simulink model "SixDOFSim"  (R2020b)
settings: Solver=VariableStepAuto  StartTime=0.0  StopTime=25  RelTol=1e-3
values from neighbouring files (symbols this model uses):
  A = q_d*S*CA    [nonlinear_6DOF.m]
  alpha_init = 0    [SixDOFModel.m]
  beta_init = 0    [SixDOFModel.m]
  eta_max = 10*pi/180    (= 0.174532925199)    [SixDOFModel.m]
  eta_min = - 25*pi/180    (= -0.436332312999)    [SixDOFModel.m]
  I_inv = inv(I)    [initializeParameters.m]
  K = place(A,B,ew_contr)    [SixDOFModel.m]
  m = 120000    [initializeParameters.m]
  Omega_init = [0;0;0]    [SixDOFModel.m]
  P_e_init = [100;0;-2000]    [SixDOFModel.m]
  Phi_init = [0;0;0]    [SixDOFModel.m]
  q = X(2)    [nonlinear_6DOF.m]
  r = X(5)    [nonlinear_6DOF.m]
  sigmaf_max = 10*pi/180    (= 0.174532925199)    [SixDOFModel.m]
  sigmaf_min = 0.5*pi/180    (= 0.00872664625997)    [SixDOFModel.m]
  U_test = [0.5;1;0;0]    [SixDOFModel.m]
  V_init = [20;0;0]    [SixDOFModel.m]
  vA_init = sqrt(V_init(1)^2+V_init(2)^2+V_init(3)^2)    [SixDOFModel.m]
  X_init = [alpha_init;Omega_init(2);vA_init;Phi_init(2);Omega_init(3);beta_init;Omega_init(1);Phi_init(1); P_e_init(1);P_e_init(2);P_e_init(3);Phi_init(3);V_init]    [SixDOFModel.m]
  xi_max = 25*pi/180    (= 0.436332312999)    [SixDOFModel.m]
  xi_min = - xi_max    (= -0.436332312999)    [SixDOFModel.m]
  zita_max = 30*pi/180    (= 0.523598775598)    [SixDOFModel.m]
  zita_min = - zita_max    (= -0.523598775598)    [SixDOFModel.m]
undefined symbols (not defined in the file or in its folder): B, Earth, F, Light, MIL, nonlinear_6DOF, WGS84
libraries: aerolibfltsims x5, aerolibtransform2 x4, aerolibwind2 x1, aerolibatmos2 x1
settings Model: Creator=teteu  LastModifiedBy=teteu
settings SolverCC: ZeroCrossAlgorithm=Adaptive
settings DebuggingCC: IgnoredZcDiagnostic=none

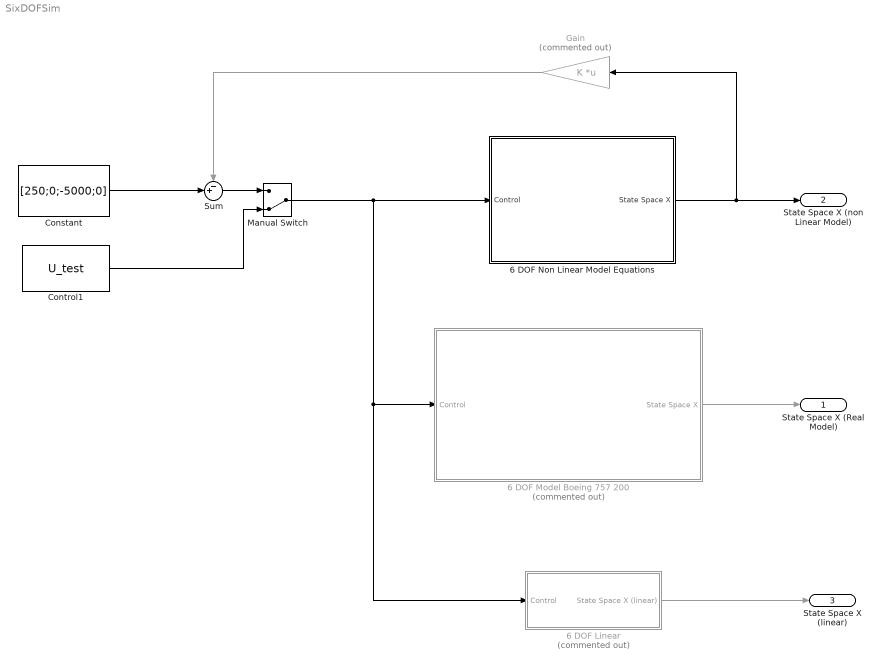
== system SixDOFSim ==
  6 DOF Linear : Subsystem  Commented=on
  6 DOF Model Boeing 757 200 : Subsystem  Commented=on
      mask Display: image('Eastern_Airlines_Boeing_757-225_N523EA_March_1990_DCW_4974892113-624x422.jpg'); % Use "Edit Image" on toolstrip to change.
  6 DOF Non Linear Model Equations : Subsystem
  Constant : Constant  Value=[250;0;-5000;0]
  Control1 : Constant  Value=U_test
  Gain : Gain  Commented=on  Gain=K  Multiplication=Matrix(K*u)
  Manual Switch : ManualSwitch  CurrentSetting=0
  Sum : Sum  Inputs=-+|
  State Space X (Real Model) : Outport
  State Space X (non Linear Model) : Outport  Port=2
  State Space X (linear) : Outport  Port=3
  wires:
  6 DOF Model Boeing 757 200/1(State Space X) -> State Space X (Real Model)/1
  6 DOF Non Linear Model Equations/1(State Space X) -> Gain/1, State Space X (non Linear Model)/1
  6 DOF Linear/1(State Space X (linear)) -> State Space X (linear)/1
  Gain/1 -> Sum/1
  Constant/1 -> Sum/2
  Sum/1 -> Manual Switch/1
  Control1/1 -> Manual Switch/2
  Manual Switch/1 -> 6 DOF Linear/1(Control), 6 DOF Model Boeing 757 200/1(Control), 6 DOF Non Linear Model Equations/1(Control)

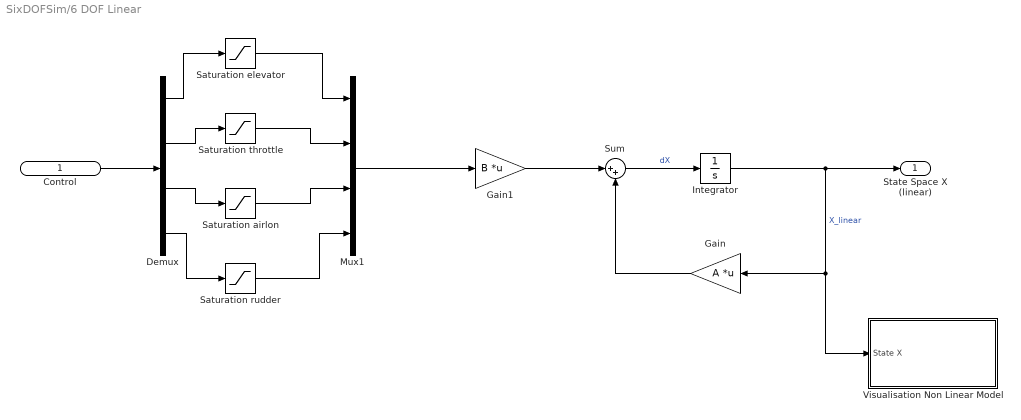
== system SixDOFSim/6 DOF Linear ==
  Control : Inport
  Demux : Demux
  Gain : Gain  Gain=A  Multiplication=Matrix(K*u)
  Gain1 : Gain  Gain=B  Multiplication=Matrix(K*u)
  Integrator : Integrator  InitialCondition=X_init
  Mux1 : Mux
  Saturation airlon : Saturate  UpperLimit=xi_max  LowerLimit=xi_min
  Saturation elevator : Saturate  UpperLimit=eta_max  LowerLimit=eta_min
  Saturation rudder : Saturate  UpperLimit=zita_max  LowerLimit=zita_min
  Saturation throttle : Saturate  UpperLimit=sigmaf_max  LowerLimit=sigmaf_min
  Sum : Sum  Inputs=|++
  Visualisation Non Linear Model : Subsystem
  State Space X (linear) : Outport
  wires:
  Gain1/1 -> Sum/1
  Integrator/1 -> State Space X (linear)/1, Visualisation Non Linear Model/1(State X), Gain/1  "X_linear"
  Mux1/1 -> Gain1/1
  Sum/1 -> Integrator/1  "dX"
  Gain/1 -> Sum/2
  Demux/2 -> Saturation throttle/1
  Demux/3 -> Saturation airlon/1
  Demux/1 -> Saturation elevator/1
  Control/1 -> Demux/1
  Saturation elevator/1 -> Mux1/1
  Saturation throttle/1 -> Mux1/2
  Saturation airlon/1 -> Mux1/3
  Saturation rudder/1 -> Mux1/4
  Demux/4 -> Saturation rudder/1

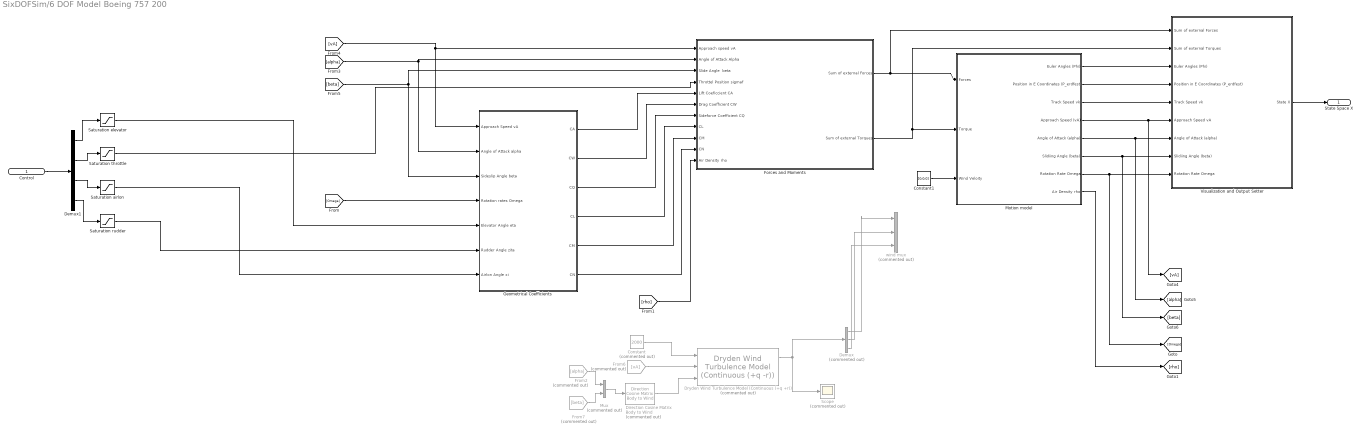
== system SixDOFSim/6 DOF Model Boeing 757 200 ==
  Control : Inport
  Constant : Constant  Commented=on  Value=2000
  Constant1 : Constant  Value=[0;0;0]
  Demux : Demux  Commented=on  Outputs=3
  Demux1 : Demux
  Direction Cosine Matrix Body to Wind : aerolibtransform2/Direction Cosine Matrix Body to Wind  Commented=on
      settings: SourceProductBaseCode=AE
  Dryden Wind Turbulence Model (Continuous (+q +r)) : aerolibwind2/Dryden Wind Turbulence Model  (Continuous (+q -r))  Commented=on  units=Metric (MKS)  spec=MIL-F-8785C  model=Continuous Dryden (+q +r)  W20=15  Wdeg=0  TurbProb=10^-2 - Light  L_high=533.4  Wingspan=10  ts=0.1  Seed=[23341 23342 23343 23344]  T_on=on
  Forces and Moments : Subsystem
  From2 : From  Commented=on  GotoTag=alpha
  From6 : From  Commented=on  GotoTag=vA
  From7 : From  Commented=on  GotoTag=beta
  Geometrical Coefficients : Subsystem
  "Motion model " : Subsystem
  Mux : Mux  Commented=on  Inputs=2
  Saturation airlon : Saturate  UpperLimit=xi_max  LowerLimit=xi_min
  Saturation elevator : Saturate  UpperLimit=eta_max  LowerLimit=eta_min
  Saturation rudder : Saturate  UpperLimit=zita_max  LowerLimit=zita_min
  Saturation throttle : Saturate  UpperLimit=sigmaf_max  LowerLimit=sigmaf_min
  Scope : Scope  Commented=on
  Visualization and Output Setter : Subsystem
  wind mux : Mux  Commented=on  Inputs=3
  State Space X : Outport
  wires:
  "Motion model "/7(Rotation Rate Omega) -> [Omega], Visualization and Output Setter/9(Rotation Rate Omega)
  "Motion model "/3(Track Speed vk) -> Visualization and Output Setter/5(Track Speed vk)
  Dryden Wind Turbulence Model (Continuous (+q +r))/1 -> Scope/1, Demux/1
  Visualization and Output Setter/1(State X) -> State Space X/1
  "Motion model "/6(Slidiing Angle (beta)) -> [beta], Visualization and Output Setter/8(Slidiing Angle (beta))
  Forces and Moments/2(Sum of external Torques) -> "Motion model "/2(Torque), Visualization and Output Setter/2(Sum of external Torques)
  [alpha] -> Geometrical Coefficients/2(Angle of Attack alpha), Forces and Moments/2(Angle of Attack Alpha)
  "Motion model "/4(Approach Speed (vA)) -> [vA], Visualization and Output Setter/6(Approach Speed vA)
  Geometrical Coefficients/4(CL) -> Forces and Moments/8(CL)
  Geometrical Coefficients/1(CA) -> Forces and Moments/5(Lift Coeficcient CA)
  Forces and Moments/1(Sum of external Forces) -> Visualization and Output Setter/1(Sum of external Forces), "Motion model "/1(Forces)
  "Motion model "/5(Angle of Attack (alpha)) -> [alpha], Visualization and Output Setter/7(Angle of Attack (alpha))
  "Motion model "/2(Position in E Coordinates (P_erdfest)) -> Visualization and Output Setter/4(Position in E Coordinates (P_erdfest))
  "Motion model "/1(Euler Angles (Phi)) -> Visualization and Output Setter/3(Euler Angles (Phi))
  [vA] -> Geometrical Coefficients/1(Approach Speed vA), Forces and Moments/1(Approach speed vA)
  Geometrical Coefficients/5(CM) -> Forces and Moments/9(CM)
  Saturation airlon/1 -> Geometrical Coefficients/7(Airlon Angle xi)
  [Omega] -> Geometrical Coefficients/4(Rotation rates Omega)
  Saturation throttle/1 -> Forces and Moments/4(Throttel Position sigmaf)
  [beta] -> Geometrical Coefficients/3(Sideslip Angle beta), Forces and Moments/3(Slide Angle  beta)
  Geometrical Coefficients/6(CN) -> Forces and Moments/10(CN)
  "Motion model "/8(Air Density rho) -> [rho]
  [rho] -> Forces and Moments/11(Air Density rho)
  Saturation elevator/1 -> Geometrical Coefficients/5(Elevator Angle eta)
  Saturation rudder/1 -> Geometrical Coefficients/6(Rudder Angle zita)
  Geometrical Coefficients/3(CQ) -> Forces and Moments/7(Sideforce Coefficient CQ)
  Constant/1 -> Dryden Wind Turbulence Model (Continuous (+q +r))/1
  Geometrical Coefficients/2(CW) -> Forces and Moments/6(Drag Coefficient CW)
  From6/1 -> Dryden Wind Turbulence Model (Continuous (+q +r))/2
  Demux/1 -> wind mux/1
  Demux/2 -> wind mux/2
  Demux/3 -> wind mux/3
  Direction Cosine Matrix Body to Wind/1 -> Dryden Wind Turbulence Model (Continuous (+q +r))/3
  From2/1 -> Mux/1
  From7/1 -> Mux/2
  Mux/1 -> Direction Cosine Matrix Body to Wind/1
  Constant1/1 -> "Motion model "/3(Wind Veloity)
  Demux1/2 -> Saturation throttle/1
  Demux1/3 -> Saturation airlon/1
  Demux1/1 -> Saturation elevator/1
  Control/1 -> Demux1/1
  Demux1/4 -> Saturation rudder/1

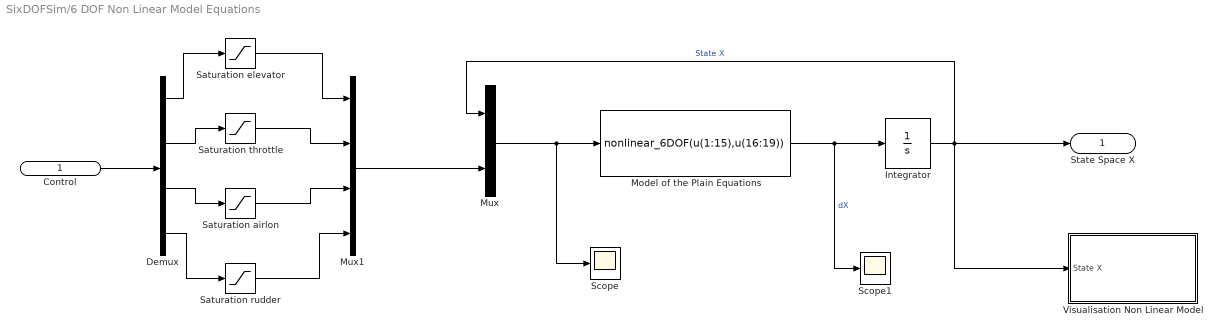
== system SixDOFSim/6 DOF Non Linear Model Equations ==
  Control : Inport
  Demux : Demux
  Integrator : Integrator  InitialCondition=X_init
  Model of the Plain Equations : MATLABFcn  MATLABFcn=nonlinear_6DOF(u(1:15),u(16:19))
  Mux : Mux  Inputs=2
  Mux1 : Mux
  Saturation airlon : Saturate  UpperLimit=xi_max  LowerLimit=xi_min
  Saturation elevator : Saturate  UpperLimit=eta_max  LowerLimit=eta_min
  Saturation rudder : Saturate  UpperLimit=zita_max  LowerLimit=zita_min
  Saturation throttle : Saturate  UpperLimit=sigmaf_max  LowerLimit=sigmaf_min
  Scope : Scope
  Scope1 : Scope
  Visualisation Non Linear Model : Subsystem
  State Space X : Outport
  wires:
  Model of the Plain Equations/1 -> Scope1/1, Integrator/1  "dX"
  Integrator/1 -> State Space X/1, Visualisation Non Linear Model/1(State X), Mux/1  "State X"
  Mux/1 -> Scope/1, Model of the Plain Equations/1
  Demux/1 -> Saturation elevator/1
  Demux/2 -> Saturation throttle/1
  Demux/3 -> Saturation airlon/1
  Demux/4 -> Saturation rudder/1
  Saturation elevator/1 -> Mux1/1
  Saturation throttle/1 -> Mux1/2
  Saturation airlon/1 -> Mux1/3
  Saturation rudder/1 -> Mux1/4
  Mux1/1 -> Mux/2
  Control/1 -> Demux/1

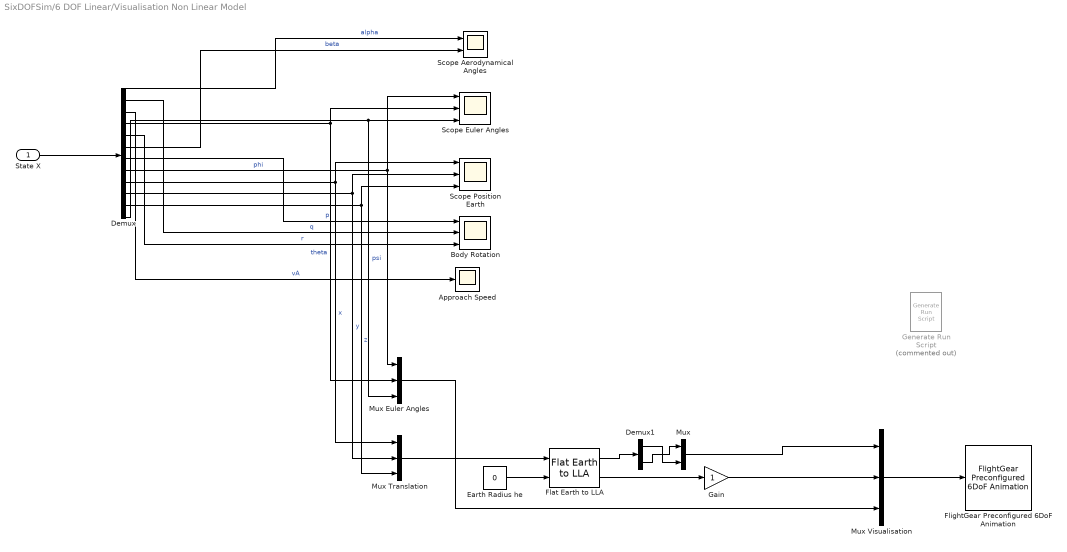
== system SixDOFSim/6 DOF Linear/Visualisation Non Linear Model ==
  State X : Inport
  Approach Speed : Scope
  Body Rotation : Scope  NumInputPorts=3
  Demux : Demux  Outputs=12
  Demux1 : Demux  Outputs=2
  Earth Radius he : Constant  Value=0
  Flat Earth to LLA : aerolibtransform2/Flat Earth to LLA  units=Metric (MKS)  ptype=Earth (WGS84)  F=1/298.257223563  R=6378137  refPosPort=off  LL0=[0 10]  psi=0
  FlightGear Preconfigured 6DoF Animation : aerolibfltsims/FlightGear Preconfigured 6DoF Animation  xFlightGearVersion=v2019.1  DestinationIpAddress=127.0.0.1  DestinationPort=5502  SampleTime=1/30  packetVersion=24
  Gain : Gain
  Generate Run Script : aerolibfltsims/Generate Run Script  Commented=on  Architecture=Win64  dataFlow=Send  GeometryModelName=c172p  AirportId=KSFO  RunwayId=10L  InitialAltitude=7224  InitialHeading=113  OffsetDistance=4.72  OffsetAzimuth=0  InstallScenery=off  DisableShaders=on  OriginAddress=127.0.0.1  DestinationPort=5502  OriginPort=5505  LocalAddress=127.0.0.1  OutputFileName=runfg.bat  FlightGearBaseDirectory=D:\Flight Gear\FlightGear 2018.1.1
  Mux : Mux  Inputs=2
  Mux Euler Angles : Mux  Inputs=3
  "Mux Translation " : Mux  Inputs=3
  Mux Visualisation : Mux  Inputs=3
  Scope Aerodynamical Angles : Scope  NumInputPorts=2
  Scope Euler Angles : Scope  NumInputPorts=3
  Scope Position Earth : Scope  NumInputPorts=3
  wires:
  Demux/4 -> Mux Euler Angles/2, Scope Euler Angles/2  "theta"
  Demux/10 -> Scope Position Earth/2, "Mux Translation "/2  "y"
  Demux/7 -> Body Rotation/1  "p"
  Demux/12 -> Scope Euler Angles/3, Mux Euler Angles/3  "psi"
  Demux/9 -> "Mux Translation "/1, Scope Position Earth/1  "x"
  Demux/8 -> Mux Euler Angles/1, Scope Euler Angles/1  "phi"
  Demux/6 -> Scope Aerodynamical Angles/2  "beta"
  Demux/3 -> Approach Speed/1  "vA"
  Demux/11 -> Scope Position Earth/3, "Mux Translation "/3  "z"
  Demux/1 -> Scope Aerodynamical Angles/1  "alpha"
  Demux/2 -> Body Rotation/2  "q"
  Demux/5 -> Body Rotation/3  "r"
  State X/1 -> Demux/1
  Earth Radius he/1 -> Flat Earth to LLA/2
  "Mux Translation "/1 -> Flat Earth to LLA/1
  Mux Visualisation/1 -> FlightGear Preconfigured 6DoF Animation/1
  Flat Earth to LLA/1 -> Demux1/1
  Demux1/1 -> Mux/2
  Demux1/2 -> Mux/1
  Mux/1 -> Mux Visualisation/1
  Mux Euler Angles/1 -> Mux Visualisation/3
  Gain/1 -> Mux Visualisation/2
  Flat Earth to LLA/2 -> Gain/1

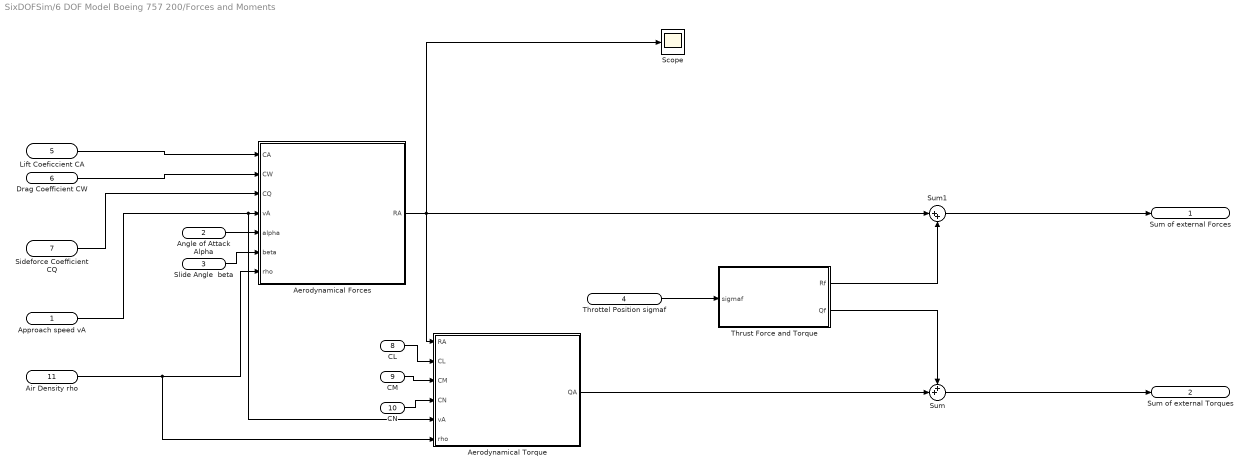
== system SixDOFSim/6 DOF Model Boeing 757 200/Forces and Moments ==
  Approach speed vA : Inport
  Angle of Attack Alpha : Inport  Port=2
  Slide Angle  beta : Inport  Port=3
  Throttel Position sigmaf : Inport  Port=4
  Lift Coeficcient CA : Inport  Port=5
  Drag Coefficient CW : Inport  Port=6
  Sideforce Coefficient CQ : Inport  Port=7
  CL : Inport  Port=8
  CM : Inport  Port=9
  CN : Inport  Port=10
  Air Density rho : Inport  Port=11
  Aerodynamical Forces : MATLAB Function  TreatAsAtomicUnit=on
  Aerodynamical Torque : MATLAB Function  TreatAsAtomicUnit=on
  Scope : Scope
  Sum : Sum  Inputs=++|
  Sum1 : Sum  Inputs=|++
  Thrust Force and Torque : MATLAB Function  TreatAsAtomicUnit=on
  Sum of external Forces : Outport
  Sum of external Torques : Outport  Port=2
  wires:
  Aerodynamical Forces/1(RA) -> Scope/1, Sum1/1, Aerodynamical Torque/1(RA)
  Aerodynamical Torque/1(QA) -> Sum/2
  Sum1/1 -> Sum of external Forces/1
  Sum/1 -> Sum of external Torques/1
  Throttel Position sigmaf/1 -> Thrust Force and Torque/1(sigmaf)
  Thrust Force and Torque/1(Rf) -> Sum1/2
  Thrust Force and Torque/2(Qf) -> Sum/1
  Angle of Attack Alpha/1 -> Aerodynamical Forces/5(alpha)
  Slide Angle  beta/1 -> Aerodynamical Forces/6(beta)
  Approach speed vA/1 -> Aerodynamical Torque/5(vA), Aerodynamical Forces/4(vA)
  Lift Coeficcient CA/1 -> Aerodynamical Forces/1(CA)
  Drag Coefficient CW/1 -> Aerodynamical Forces/2(CW)
  Sideforce Coefficient CQ/1 -> Aerodynamical Forces/3(CQ)
  CL/1 -> Aerodynamical Torque/2(CL)
  CM/1 -> Aerodynamical Torque/3(CM)
  CN/1 -> Aerodynamical Torque/4(CN)
  Air Density rho/1 -> Aerodynamical Torque/6(rho), Aerodynamical Forces/7(rho)

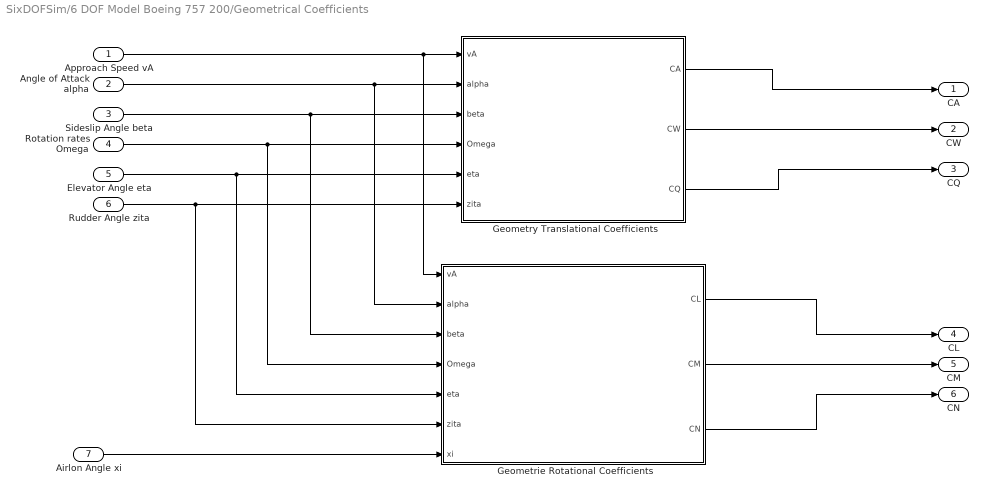
== system SixDOFSim/6 DOF Model Boeing 757 200/Geometrical Coefficients ==
  Approach Speed vA : Inport
  Angle of Attack alpha : Inport  Port=2
  Sideslip Angle beta : Inport  Port=3
  Rotation rates Omega : Inport  Port=4
  Elevator Angle eta : Inport  Port=5
  Rudder Angle zita : Inport  Port=6
  Airlon Angle xi : Inport  Port=7
  Geometrie Rotational Coefficients : MATLAB Function  TreatAsAtomicUnit=on
  Geometry Translational Coefficients : MATLAB Function  TreatAsAtomicUnit=on
  CA : Outport
  CW : Outport  Port=2
  CQ : Outport  Port=3
  CL : Outport  Port=4
  CM : Outport  Port=5
  CN : Outport  Port=6
  wires:
  Elevator Angle eta/1 -> Geometrie Rotational Coefficients/5(eta), Geometry Translational Coefficients/5(eta)
  Angle of Attack alpha/1 -> Geometrie Rotational Coefficients/2(alpha), Geometry Translational Coefficients/2(alpha)
  Geometrie Rotational Coefficients/1(CL) -> CL/1
  Geometry Translational Coefficients/3(CQ) -> CQ/1
  Geometrie Rotational Coefficients/3(CN) -> CN/1
  Approach Speed vA/1 -> Geometrie Rotational Coefficients/1(vA), Geometry Translational Coefficients/1(vA)
  Geometry Translational Coefficients/1(CA) -> CA/1
  Sideslip Angle beta/1 -> Geometrie Rotational Coefficients/3(beta), Geometry Translational Coefficients/3(beta)
  Rudder Angle zita/1 -> Geometrie Rotational Coefficients/6(zita), Geometry Translational Coefficients/6(zita)
  Geometry Translational Coefficients/2(CW) -> CW/1
  Rotation rates Omega/1 -> Geometrie Rotational Coefficients/4(Omega), Geometry Translational Coefficients/4(Omega)
  Geometrie Rotational Coefficients/2(CM) -> CM/1
  Airlon Angle xi/1 -> Geometrie Rotational Coefficients/7(xi)

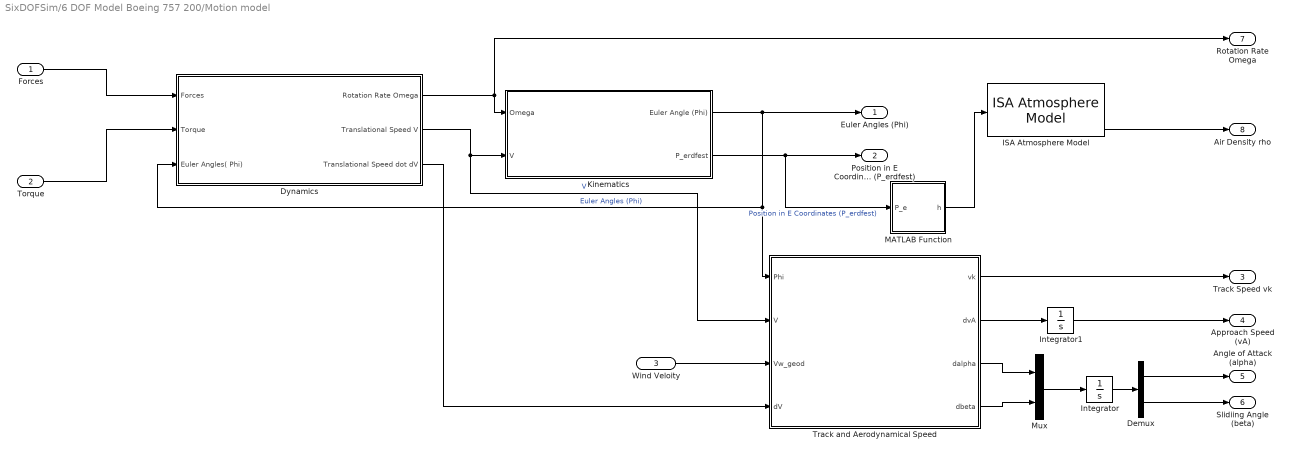
== system SixDOFSim/6 DOF Model Boeing 757 200/Motion model  ==
  Forces : Inport
  Torque : Inport  Port=2
  Wind Veloity : Inport  Port=3
  Demux : Demux  Outputs=2
  Dynamics : Subsystem
  ISA Atmosphere Model : aerolibatmos2/ISA Atmosphere Model  custom=off  g=9.80665  gamma=1.4  R=287.0531  L=0.0065  h_trop=11000  h_strat=20000  rho0=1.225  P0=101325  T0=288.15  h0=0
  Integrator : Integrator  InitialCondition=[alpha_init;beta_init]
  Integrator1 : Integrator  InitialCondition=vA_init
  Kinematics : Subsystem
  MATLAB Function : MATLAB Function  TreatAsAtomicUnit=on
  Mux : Mux  Inputs=2
  Track and Aerodynamical Speed : MATLAB Function  TreatAsAtomicUnit=on
  Euler Angles (Phi) : Outport
  Position in E Coordinates (P_erdfest) : Outport  Port=2
  Track Speed vk : Outport  Port=3
  Approach Speed (vA) : Outport  Port=4
  Angle of Attack (alpha) : Outport  Port=5
  Slidiing Angle (beta) : Outport  Port=6
  Rotation Rate Omega : Outport  Port=7
  Air Density rho : Outport  Port=8
  wires:
  Torque/1 -> Dynamics/2(Torque)
  Kinematics/1(Euler Angle (Phi)) -> Track and Aerodynamical Speed/1(Phi), Dynamics/3(Euler Angles( Phi)), Euler Angles (Phi)/1  "Euler Angles (Phi)"
  Kinematics/2(P_erdfest) -> Position in E Coordinates (P_erdfest)/1, MATLAB Function/1(P_e)  "Position in E Coordinates (P_erdfest)"
  Dynamics/2(Translational Speed V) -> Track and Aerodynamical Speed/2(V), Kinematics/2(V)  "V"
  Forces/1 -> Dynamics/1(Forces)
  Dynamics/1(Rotation Rate Omega) -> Kinematics/1(Omega), Rotation Rate Omega/1
  Wind Veloity/1 -> Track and Aerodynamical Speed/3(Vw_geod)
  MATLAB Function/1(h) -> ISA Atmosphere Model/1
  ISA Atmosphere Model/4 -> Air Density rho/1
  Track and Aerodynamical Speed/1(vk) -> Track Speed vk/1
  Dynamics/3(Translational Speed dot dV) -> Track and Aerodynamical Speed/4(dV)
  Mux/1 -> Integrator/1
  Integrator/1 -> Demux/1
  Demux/1 -> Angle of Attack (alpha)/1
  Demux/2 -> Slidiing Angle (beta)/1
  Track and Aerodynamical Speed/3(dalpha) -> Mux/1
  Track and Aerodynamical Speed/4(dbeta) -> Mux/2
  Track and Aerodynamical Speed/2(dvA) -> Integrator1/1
  Integrator1/1 -> Approach Speed (vA)/1

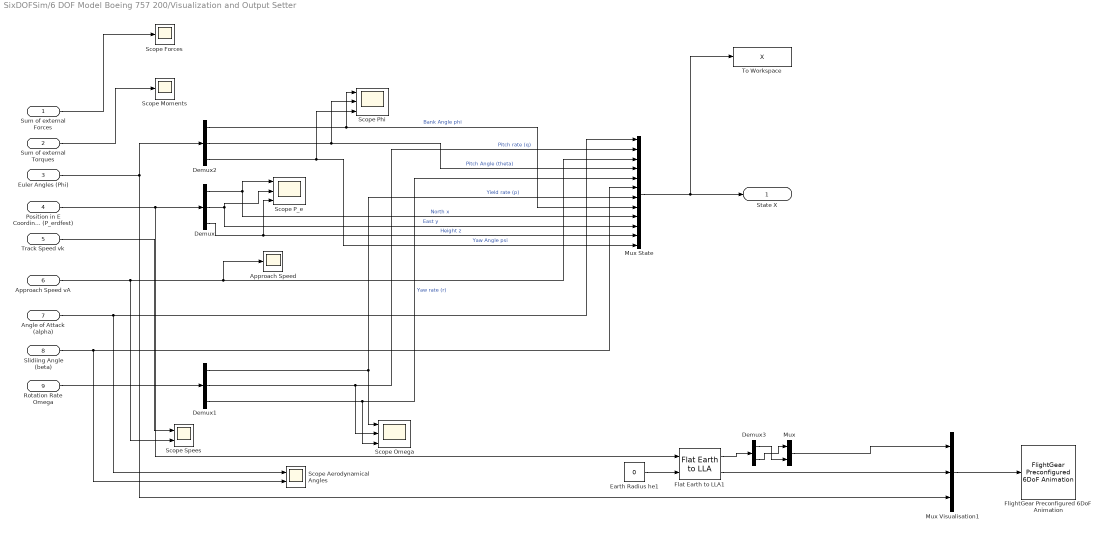
== system SixDOFSim/6 DOF Model Boeing 757 200/Visualization and Output Setter ==
  Sum of external Forces : Inport
  Sum of external Torques : Inport  Port=2
  Euler Angles (Phi) : Inport  Port=3
  Position in E Coordinates (P_erdfest) : Inport  Port=4
  Track Speed vk : Inport  Port=5
  Approach Speed vA : Inport  Port=6
  Angle of Attack (alpha) : Inport  Port=7
  Slidiing Angle (beta) : Inport  Port=8
  Rotation Rate Omega : Inport  Port=9
  Approach Speed : Scope
  Demux : Demux  Outputs=3
  Demux1 : Demux  Outputs=3
  Demux2 : Demux  Outputs=3
  Demux3 : Demux  Outputs=2
  Earth Radius he1 : Constant  Value=0
  Flat Earth to LLA1 : aerolibtransform2/Flat Earth to LLA  units=Metric (MKS)  ptype=Earth (WGS84)  F=1/298.257223563  R=6378137  refPosPort=off  LL0=[0 10]  psi=0
  FlightGear Preconfigured 6DoF Animation : aerolibfltsims/FlightGear Preconfigured 6DoF Animation  xFlightGearVersion=v2019.1  DestinationIpAddress=127.0.0.1  DestinationPort=5502  SampleTime=1/30  packetVersion=24
  Mux : Mux  Inputs=2
  Mux State : Mux  Inputs=12
  Mux Visualisation1 : Mux  Inputs=3
  Scope Aerodynamical Angles : Scope  NumInputPorts=2
  Scope Forces : Scope
  Scope Moments : Scope
  Scope Omega : Scope  NumInputPorts=3
  Scope P_e : Scope  NumInputPorts=3
  Scope Phi : Scope  NumInputPorts=3
  Scope Spees : Scope  NumInputPorts=2
  To Workspace : ToWorkspace  VariableName=X  SaveFormat=Timeseries  SampleTime=-1
  State X : Outport
  wires:
  Rotation Rate Omega/1 -> Demux1/1
  Position in E Coordinates (P_erdfest)/1 -> Demux/1, Flat Earth to LLA1/1
  Mux State/1 -> To Workspace/1, State X/1
  Angle of Attack (alpha)/1 -> Mux State/1, Scope Aerodynamical Angles/1
  Demux1/2 -> Mux State/2, Scope Omega/2  "Pitch rate (q)"
  Approach Speed vA/1 -> Scope Spees/2, Approach Speed/1, Mux State/3
  Euler Angles (Phi)/1 -> Demux2/1, Mux Visualisation1/3
  Demux2/2 -> Mux State/4, Scope Phi/2  "Pitch Angle (theta)"
  Demux1/3 -> Mux State/5, Scope Omega/3  "Yaw rate (r)"
  Slidiing Angle (beta)/1 -> Mux State/6, Scope Aerodynamical Angles/2
  Demux1/1 -> Scope Omega/1, Mux State/7  "Yield rate (p)"
  Demux2/1 -> Scope Phi/1, Mux State/8  "Bank Angle phi"
  Demux/1 -> Scope P_e/1, Mux State/9  "North x"
  Demux/2 -> Scope P_e/2, Mux State/10  "East y"
  Demux/3 -> Scope P_e/3, Mux State/11  "Height z"
  Demux2/3 -> Mux State/12, Scope Phi/3  "Yaw Angle psi"
  Sum of external Forces/1 -> Scope Forces/1
  Sum of external Torques/1 -> Scope Moments/1
  Track Speed vk/1 -> Scope Spees/1
  Demux3/1 -> Mux/2
  Flat Earth to LLA1/2 -> Mux Visualisation1/2
  Demux3/2 -> Mux/1
  Mux Visualisation1/1 -> FlightGear Preconfigured 6DoF Animation/1
  Flat Earth to LLA1/1 -> Demux3/1
  Earth Radius he1/1 -> Flat Earth to LLA1/2
  Mux/1 -> Mux Visualisation1/1

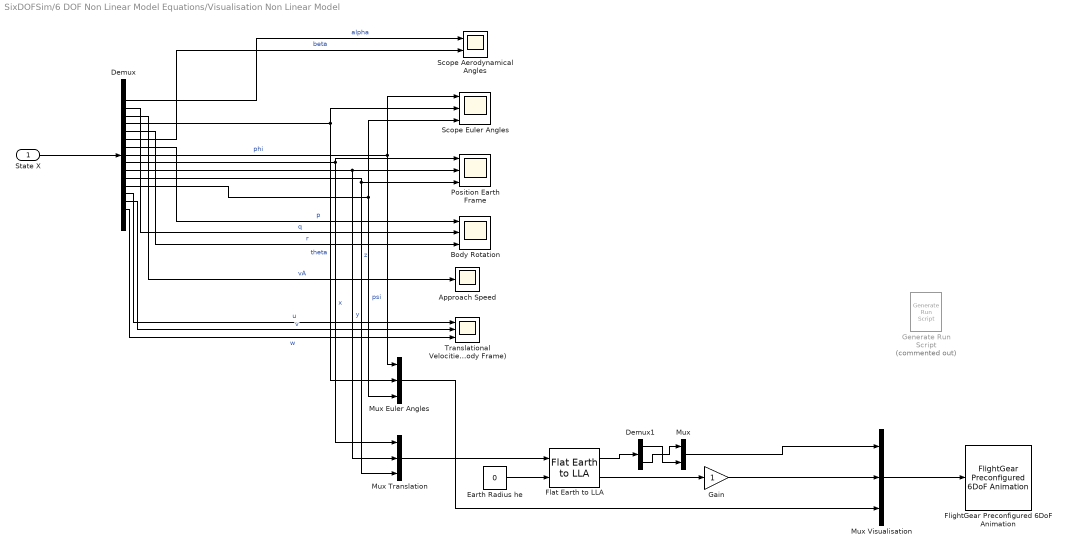
== system SixDOFSim/6 DOF Non Linear Model Equations/Visualisation Non Linear Model ==
  State X : Inport
  Approach Speed : Scope
  Body Rotation : Scope  NumInputPorts=3
  Demux : Demux  Outputs=15
  Demux1 : Demux  Outputs=2
  Earth Radius he : Constant  Value=0
  Flat Earth to LLA : aerolibtransform2/Flat Earth to LLA  units=Metric (MKS)  ptype=Earth (WGS84)  F=1/298.257223563  R=6378137  refPosPort=off  LL0=[0 10]  psi=0
  FlightGear Preconfigured 6DoF Animation : aerolibfltsims/FlightGear Preconfigured 6DoF Animation  xFlightGearVersion=v2019.1  DestinationIpAddress=127.0.0.1  DestinationPort=5502  SampleTime=1/30  packetVersion=24
  Gain : Gain
  Generate Run Script : aerolibfltsims/Generate Run Script  Commented=on  Architecture=Win64  dataFlow=Send  GeometryModelName=c172p  AirportId=KSFO  RunwayId=10L  InitialAltitude=7224  InitialHeading=113  OffsetDistance=4.72  OffsetAzimuth=0  InstallScenery=off  DisableShaders=on  OriginAddress=127.0.0.1  DestinationPort=5502  OriginPort=5505  LocalAddress=127.0.0.1  OutputFileName=runfg.bat  FlightGearBaseDirectory=D:\Flight Gear\FlightGear 2018.1.1
  Mux : Mux  Inputs=2
  Mux Euler Angles : Mux  Inputs=3
  "Mux Translation " : Mux  Inputs=3
  Mux Visualisation : Mux  Inputs=3
  Position Earth Frame : Scope  NumInputPorts=3
  Scope Aerodynamical Angles : Scope  NumInputPorts=2
  Scope Euler Angles : Scope  NumInputPorts=3
  Translational Velocities (Body Frame) : Scope  NumInputPorts=3
  wires:
  Demux/4 -> Mux Euler Angles/2, Scope Euler Angles/2  "theta"
  Demux/10 -> "Mux Translation "/2, Position Earth Frame/2  "y"
  Demux/7 -> Body Rotation/1  "p"
  Demux/12 -> Scope Euler Angles/3, Mux Euler Angles/3  "psi"
  Demux/9 -> "Mux Translation "/1, Position Earth Frame/1  "x"
  Demux/8 -> Mux Euler Angles/1, Scope Euler Angles/1  "phi"
  Demux/6 -> Scope Aerodynamical Angles/2  "beta"
  Demux/3 -> Approach Speed/1  "vA"
  Demux/11 -> "Mux Translation "/3, Position Earth Frame/3  "z"
  Demux/1 -> Scope Aerodynamical Angles/1  "alpha"
  Demux/2 -> Body Rotation/2  "q"
  Demux/5 -> Body Rotation/3  "r"
  State X/1 -> Demux/1
  Earth Radius he/1 -> Flat Earth to LLA/2
  "Mux Translation "/1 -> Flat Earth to LLA/1
  Mux Visualisation/1 -> FlightGear Preconfigured 6DoF Animation/1
  Flat Earth to LLA/1 -> Demux1/1
  Demux1/1 -> Mux/2
  Demux1/2 -> Mux/1
  Mux/1 -> Mux Visualisation/1
  Mux Euler Angles/1 -> Mux Visualisation/3
  Gain/1 -> Mux Visualisation/2
  Flat Earth to LLA/2 -> Gain/1
  Demux/13 -> Translational Velocities (Body Frame)/1  "u"
  Demux/14 -> Translational Velocities (Body Frame)/2  "v"
  Demux/15 -> Translational Velocities (Body Frame)/3  "w"

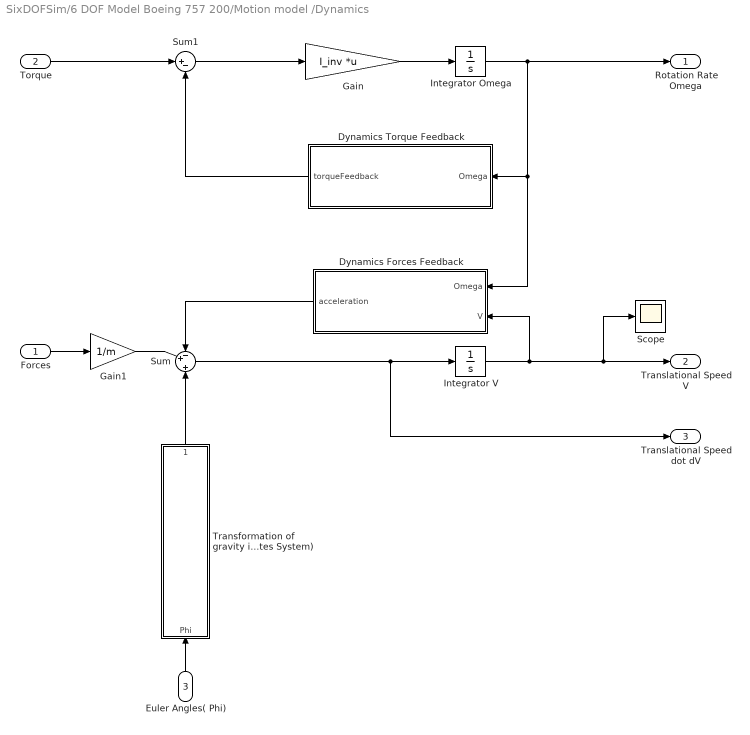
== system SixDOFSim/6 DOF Model Boeing 757 200/Motion model /Dynamics ==
  Forces : Inport
  Torque : Inport  Port=2
  Euler Angles( Phi) : Inport  Port=3
  Dynamics Forces Feedback : MATLAB Function  TreatAsAtomicUnit=on
  Dynamics Torque Feedback : MATLAB Function  TreatAsAtomicUnit=on
  Gain : Gain  Gain=I_inv  Multiplication=Matrix(K*u) (u vector)
  Gain1 : Gain  Gain=1/m
  Integrator Omega : Integrator  InitialCondition=Omega_init
  Integrator V : Integrator  InitialCondition=V_init
  Scope : Scope
  Sum : Sum  Inputs=-+|+
  Sum1 : Sum  Inputs=|+-
  Transformation of gravity in (Körperfestes System) : MATLAB Function  TreatAsAtomicUnit=on
  Rotation Rate Omega : Outport
  Translational Speed V : Outport  Port=2
  Translational Speed dot dV : Outport  Port=3
  wires:
  Euler Angles( Phi)/1 -> Transformation of gravity in (Körperfestes System)/1(Phi)
  Transformation of gravity in (Körperfestes System)/1(gravityAcceleration) -> Sum/3
  Forces/1 -> Gain1/1
  Sum/1 -> Translational Speed dot dV/1, Integrator V/1
  Integrator V/1 -> Scope/1, Translational Speed V/1, Dynamics Forces Feedback/2(V)
  Gain1/1 -> Sum/2
  Dynamics Forces Feedback/1(acceleration) -> Sum/1
  Torque/1 -> Sum1/1
  Sum1/1 -> Gain/1
  Gain/1 -> Integrator Omega/1
  Integrator Omega/1 -> Dynamics Forces Feedback/1(Omega), Dynamics Torque Feedback/1(Omega), Rotation Rate Omega/1
  Dynamics Torque Feedback/1(torqueFeedback) -> Sum1/2

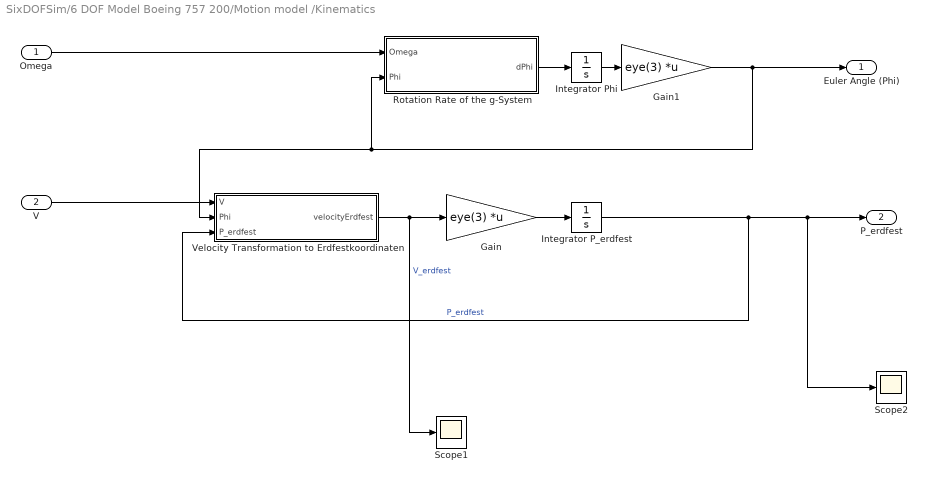
== system SixDOFSim/6 DOF Model Boeing 757 200/Motion model /Kinematics ==
  Omega : Inport
  V : Inport  Port=2
  Gain : Gain  Gain=eye(3)  Multiplication=Matrix(K*u) (u vector)
  Gain1 : Gain  Gain=eye(3)  Multiplication=Matrix(K*u) (u vector)
  Integrator P_erdfest : Integrator  InitialCondition=P_e_init
  Integrator Phi : Integrator  InitialCondition=Phi_init
  Rotation Rate of the g-System : MATLAB Function  TreatAsAtomicUnit=on
  Scope1 : Scope
  Scope2 : Scope
  Velocity Transformation to Erdfestkoordinaten : MATLAB Function  TreatAsAtomicUnit=on
  Euler Angle (Phi) : Outport
  P_erdfest : Outport  Port=2
  wires:
  Integrator P_erdfest/1 -> Scope2/1, P_erdfest/1, Velocity Transformation to Erdfestkoordinaten/3(P_erdfest)  "P_erdfest"
  Velocity Transformation to Erdfestkoordinaten/1(velocityErdfest) -> Scope1/1, Gain/1  "V_erdfest"
  V/1 -> Velocity Transformation to Erdfestkoordinaten/1(V)
  Rotation Rate of the g-System/1(dPhi) -> Integrator Phi/1
  Gain/1 -> Integrator P_erdfest/1
  Omega/1 -> Rotation Rate of the g-System/1(Omega)
  Integrator Phi/1 -> Gain1/1
  Gain1/1 -> Rotation Rate of the g-System/2(Phi), Velocity Transformation to Erdfestkoordinaten/2(Phi), Euler Angle (Phi)/1

== matlab function SixDOFSim/6 DOF Model Boeing 757 200/Motion model /Dynamics/Transformation of gravity in (Körperfestes System) ==
  data: Phi input; gravityAcceleration output; g parameter
function gravityAcceleration = Tfg(Phi,g)
G_geod = [0;0;g]; %Graviation vector in geodetic ref. Frame
Tfg = coordTransfMatrix(Phi(1),1)*coordTransfMatrix(Phi(2),2)*coordTransfMatrix(Phi(3),3); % Transformation Matrix goedetic --> body reference Frame
gravityAcceleration = Tfg*G_geod;

== matlab function SixDOFSim/6 DOF Model Boeing 757 200/Motion model /Kinematics/Rotation Rate of the g-System ==
  data: Omega input; dPhi output; Phi input
function dPhi = J(Omega,Phi)
%Rotation rate of the g-system depending on the euler angles
%Phi: euler Angles
%Omega_ diff = Omega-Omega_g
%dPhi: Rotaion Speed considering the rotation rate of the geodathic system
phi = Phi(1);
theta = Phi(2);
J = 1/cos(theta)*[cos(theta) sin(phi)*sin(theta) cos(phi)*sin(theta) ;0 cos(phi)*cos(theta) -sin(phi)*cos(theta);0 sin(phi) cos(phi)]; %Rotation rate matrix
dPhi = J*Omega;

== matlab function SixDOFSim/6 DOF Model Boeing 757 200/Motion model /Kinematics/Velocity Transformation to Erdfestkoordinaten ==
  data: V input; Phi input; velocityErdfest output; P_erdfest input
function velocityErdfest = Tef(V,Phi,P_erdfest)
%Converts the velocity from Körper to Erdfest Koordinaten
%Phi: Vector w. Euler Angles
% P_erdfest: Position Vector 
lambda = atan2(P_erdfest(2),P_erdfest(1)); %Angle Längengrad
sigma = asin(P_erdfest(3)/sqrt(P_erdfest(1)^2+P_erdfest(2)^2+P_erdfest(3)^2)); %Declination Angle 
TgE = coordTransfMatrix(-pi/2 - sigma,2)*coordTransfMatrix(lambda,3);
Tfg = coordTransfMatrix(Phi(1),1)*coordTransfMatrix(Phi(2),2)*coordTransfMatrix(Phi(3),3); % Transformation Matrix goedetic --> body reference Frame
TfE = Tfg*TgE;
TEf= TfE';
velocityErdfest = TEf*V;

== matlab function SixDOFSim/6 DOF Model Boeing 757 200/Motion model /MATLAB Function ==
  data: P_e input; h output
function h = getHeight(P_e)
h = P_e(3);

== matlab function SixDOFSim/6 DOF Model Boeing 757 200/Motion model /Track and Aerodynamical Speed ==
  data: Phi input; V input; vk output; dvA output; dalpha output; dbeta output; Vw_geod input; dV input
function [vk,dvA,dalpha,dbeta] = getTrackAndAero(Phi,V,Vw_geod,dV)
%Get The Track Speed, the Approach Speed, the inclinational angle ,
%the Azimuth angle, the angle of attack and the Sliding angle from the
%Speed from the Translational Velocity. 
Tfg = coordTransfMatrix(Phi(1),1)*coordTransfMatrix(Phi(2),2)*coordTransfMatrix(Phi(3),3); % Transformation Matrix goedetic --> body reference Frame
Tgf = Tfg';
Vk = Tgf*V; %Track Velocity
vk = sqrt(Vk(1)^2+Vk(2)^2+Vk(3)^2); %Track Speed [m/s]
%gamma = -asin(Vk(3)/vk); %Inclination Angle [rad]
%chsi = atan2(Vk(2),Vk(1));
Vw = Tfg*Vw_geod;
VA = V - Vw; %Approach Speed
vA = sqrt(VA(1)^2+VA(2)^2+VA(3)^2); %Approach Speed [m/s]
% alpha = atan(VA(3)/VA(1)); % Angle of attck [m/s]
% beta = asin(VA(2)/vA);
dvA = (VA(1)*dV(1) + VA(2)*dV(2) +VA(3)*dV(3))/(vA); %Derivative of the Approach Speed
dalpha = (dV(3)*VA(1)-dV(1)*VA(3))/(VA(1)^2+VA(1)*VA(3)); %Derivative of Angle of Attack
dbeta = (dV(2)*vA -dvA*VA(2))/(vA*sqrt(vA^2-VA(2)^2)); %Derivative of Sideslip Angle

== matlab function SixDOFSim/6 DOF Model Boeing 757 200/Geometrical Coefficients/Geometrie Rotational Coefficients ==
  data: vA input; alpha input; beta input; Omega input; eta input; zita input; globalParameters parameter; xi input; CL output; CM output; CN output
function [CL,CM,CN] = torqueGeometricCoefficient(vA,alpha,beta,Omega,eta,zita, globalParameters,xi)
%eta = Höheruderwinkel (elevator) [rad]
%zita = Seitenruderwinkel (ruder) [rad]
%xi = Querruderwinkel (Airlon) [rad]
%Global Parameters
lt = globalParameters.lt;
S = globalParameters.S;
St = globalParameters.St;
c = globalParameters.c;

%Constants Coefficients
gradient_alpha_epsolon = 0.25;
alpha_L0 = 11.5*pi/180;

epsolon = gradient_alpha_epsolon*(alpha - alpha_L0); %Downwash [rad]
N = [-1.4*beta;-0.59-3.1*(St*lt/(c*S))*(alpha-epsolon);(1-alpha*(180/(15*pi)))*beta]; %Static Moments Effects
Jakobi_CM_X = (c/vA)*[-11,    0,           5;
                      0,-4.03*St*lt^2/(S*c),0;
                      1.7,          0   , -11.5];
Jakobi_CM_U = [-0.6, 0, 0.22;
               0,    -3.1*St*lt/(S*c),0;
               0, 0, -0.63];      % Dependence of Control Variables
           
C_torque = N + Jakobi_CM_X*Omega + Jakobi_CM_U*[xi;eta;zita];
CL = C_torque(1);
CM = C_torque(2);
CN = C_torque(3);

== matlab function SixDOFSim/6 DOF Model Boeing 757 200/Geometrical Coefficients/Geometry Translational Coefficients ==
  data: vA input; alpha input; CA output; beta input; Omega input; globalParameters parameter; CW output; CQ output; eta input; zita input
function [CA,CW,CQ] = forceGeometryCoefficients(vA,alpha,beta,Omega,globalParameters,eta,zita)
%eta = Höheruderwinkel (elevator) [rad]
%zita = Seitenruderwinkel (ruder) [rad]
%Global Parameters
lt = globalParameters.lt;
S = globalParameters.S;
St = globalParameters.St;
% Rotration rates [rad/s]
q = Omega(2); %Nickrate (Pitch Rate)
%Constants Coefficients
CA0 = 1.104;
grad_alpha = 5.5;
alpha_L0 = 11.5*pi/180;
a3 = -768.5;
a2 = 609.2;
a1 = -155.2;
a0 = 15.212;
gradient_alpha_epsolon = 0.25;
gradient_CQ_Cbeta = -1.6;
gradientCQ_Czita = 0.24;
CW0 = 0.13;
kappa = 0.07;
%Geometry Coeffcients
if alpha <=14.5*pi/180
    CA_F = grad_alpha*alpha+CA0; % Lift Coefficient without the Control Aereas
else
    CA_F = a3*alpha^.3+a2*alpha^.2+a1*alpha +a0;% Lift Coefficient without the Control Aereas
end
epsolon = gradient_alpha_epsolon*(alpha - alpha_L0); %Downwash [rad]
alpha_t = alpha - epsolon + eta +q*lt/vA; %Angle of Attack of the Tail [rad]
CA_H = 3.1*(St/S)*alpha_t; %Lift Coefficient of the Control Aereas (Elevator-Tail)
CA = CA_F + CA_H; %Total Lift Coefficient
CW = CW0 + kappa*(5.5*alpha + 0.654)^2; %Drag Coefficient
CQ = gradient_CQ_Cbeta*beta + gradientCQ_Czita*zita;

== matlab function SixDOFSim/6 DOF Model Boeing 757 200/Forces and Moments/Aerodynamical Forces ==
  data: CA input; RA output; CW input; CQ input; vA input; alpha input; beta input; rho input; globalParameters parameter
function RA = getAerodynForces(CA,CW,CQ,vA, alpha, beta, rho,globalParameters)
%[~,~,~,rho] = atmosisa(h); %Air density 
q_d = 0.5*vA^2*rho; %Dynamic Preassure
S = globalParameters.S ;


A = q_d*S*CA; %Lift Force [N]
W = q_d*S*CW; %Air Resistance [N]
Q = q_d*S*CQ; %Transverse Force [N]

Tfa = coordTransfMatrix(alpha,2)*coordTransfMatrix(-beta,3); %Transformation Matrix Aerodynamics -> Körperfest

RA_a =[-W;Q;-A];
RA = Tfa*RA_a;

== matlab function SixDOFSim/6 DOF Model Boeing 757 200/Forces and Moments/Aerodynamical Torque ==
  data: RA input; CL input; QA output; CM input; CN input; vA input; globalParameters parameter; rho input
function QA = getAerodynTorque(RA,CL,CM,CN, vA, globalParameters,rho)
% h = P_e(3); %Height [m]
% [~,~,~,rho] = atmosisa(h); %Air density 
%Aircraft Parameters
b = globalParameters.b;
%rho = globalParameters.rho;
c = globalParameters.c;
S = globalParameters.S;
P_centerGravity = globalParameters.P_centerGravity;
P_aerodynCenter = globalParameters.P_aerodynCenter;
q_d = 0.5*vA^2*rho; %Dynamic Preassure


QA_aerodynCenter = q_d*S*[0.5*b*CL;c*CM;0.5*b*CN];
QA = QA_aerodynCenter + vecToMat(P_centerGravity- P_aerodynCenter)*RA;

== matlab function SixDOFSim/6 DOF Model Boeing 757 200/Forces and Moments/Thrust Force and Torque ==
  data: sigmaf input; Rf output; globalParameters parameter; Qf output
function [Rf,Qf] = thrust(sigmaf,globalParameters)
%Get Thrus Force Rf and Thrust Moment Qf
%sigmaf: Throttle Position [rad]
P_thrust =globalParameters.P_thrust;
i_f =globalParameters.i_f;
F_max = globalParameters.Fmax;

F_res = F_max*sigmaf; %Resultant Force Absolute Value
Rf = F_res*[cos(i_f);0;sin(i_f)]; %Thrust Force 
P_thrust_tilde = vecToMat(P_thrust);
Qf = P_thrust_tilde*Rf; %Thrust Moment

== matlab function SixDOFSim/6 DOF Model Boeing 757 200/Motion model /Dynamics/Dynamics Forces Feedback ==
  data: Omega input; V input; acceleration output; globalParameters parameter
function acceleration = accelerationFeedback(Omega,V,globalParameters)
Omega_e_tilde = globalParameters.Omega_e_tilde;
Omega_tilde = vecToMat(Omega);
acceleration = (Omega_tilde + Omega_e_tilde)*V;

== matlab function SixDOFSim/6 DOF Model Boeing 757 200/Motion model /Dynamics/Dynamics Torque Feedback ==
  data: Omega input; torqueFeedback output; globalParameters parameter
function torqueFeedback = getTorqueFeedback(Omega,globalParameters)
I = globalParameters.I;
Omega_tilde = vecToMat(Omega);
help = Omega_tilde*I;
torqueFeedback = help*Omega;
